simulink model "WBFM"  (R2021a)
settings: Solver=FixedStepAuto  StartTime=0.0  StopTime=10.0  RelTol=1e-3
libraries: dspsrcs4 x1
settings Model: Creator=Bharat Gunhalkar  LastModifiedBy=Bharat Gunhalkar

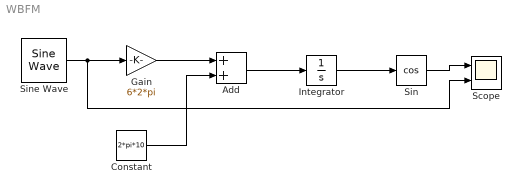
== system WBFM ==
  Add : Sum
  Constant : Constant  Value=2*pi*10
  Gain : Gain  Gain=6*2*pi
  Integrator : Integrator
  Scope : Scope  NumInputPorts=2
  Sin : Trigonometry  Operator=cos
  Sine Wave : dspsrcs4/Sine Wave  Amplitude=1  Frequency=2*pi  Phase=pi/2  SampleMode=Discrete  OutComplex=Real  CompMethod=Trigonometric fcn  TableSize=Speed  SampleTime=1/1000  SamplesPerFrame=1  ResetState=Restart at time zero  OutputFrames=off  dataType=double  wordLen=16  udDataType=sfix(16)  fracBitsMode=Best precision  numFracBits=15  OutDataTypeStr=double  LastOutDataTypeStr=double
  wires:
  Sine Wave/1 -> Scope/2, Gain/1
  Constant/1 -> Add/2
  Gain/1 -> Add/1
  Sin/1 -> Scope/1
  Integrator/1 -> Sin/1
  Add/1 -> Integrator/1
